simulink model "bdot_dynamic_test"  (R2016b)
settings: Solver=ode23tb  StartTime=0.0  StopTime=1000  RelTol=1e-3  EnableMultiTasking=on
libraries: dynamics_lib x1, environment_lib x1, bdot_controller_lib x1, command_processing x1, magnetometer_lib x1, magnetorquer_assembly_lib x1
settings Model: Creator=Taylor  LastModifiedBy=Taylor
settings OptimizationCC: DefaultParameterBehavior=Inlined  UseDivisionForNetSlopeComputation=on  UseFloatMulNetSlope=on  InlineInvariantSignals=on  PassReuseOutputArgsAs=Individual arguments  ZeroExternalMemoryAtStartup=off  ZeroInternalMemoryAtStartup=off  NoFixptDivByZeroProtection=on  EfficientFloat2IntCast=on  LifeSpan=1
settings DebuggingCC: ParameterTunabilityLossMsg=error  SFUnexpectedBacktrackingDiag=warning  SFNoUnconditionalDefaultTransitionDiag=warning  SFExecutionAtInitializationDiag=none
settings HardwareCC: ProdBitPerInt=16  ProdBitPerPointer=16  ProdBitPerSizeT=16  ProdBitPerPtrDiffT=16  ProdLargestAtomicFloat=None  ProdWordSize=16  ProdHWDeviceType=Texas Instruments->MSP430
settings RTWCC: SystemTargetFile=ert.tlc  TemplateMakefile=ert_default_tmf  Description=Embedded Coder  GenerateReport=on  IncludeHyperlinkInReport=on  LaunchReport=on  GenerateTraceInfo=on  GenerateTraceReport=on  GenerateTraceReportSl=on  GenerateTraceReportSf=on  GenerateTraceReportEml=on  GenerateCodeMetricsReport=on
settings CodeAppCC: ForceParamTrailComments=on  IgnoreCustomStorageClasses=off  OperatorAnnotations=on  SimulinkDataObjDesc=on  SFDataObjDesc=on  MATLABFcnDesc=on  CustomSymbolStrGlobalVar=rt$N$M  CustomSymbolStrType=$N$M  CustomSymbolStrFcn=$N$M$F  CustomSymbolStrMacro=$N$M  InsertBlockDesc=on  MATLABSourceComments=on
settings ERTTargetCC: GenerateSampleERTMain=on  CombineSignalStateStructs=on  SupportComplex=off  SupportContinuousTime=on  SupportNonInlinedSFcns=on  InlinedParameterPlacement=NonHierarchical  ERTCustomFileTemplate=example_file_process.tlc  ERTFilePackagingFormat=CompactWithDataFile
settings ConfigComp: CovMetricSettings=dw  CovHtmlReporting=on  CovSaveCumulativeToWorkspaceVar=on  CovSaveSingleToWorkspaceVar=on  CovExternalEMLEnable=off

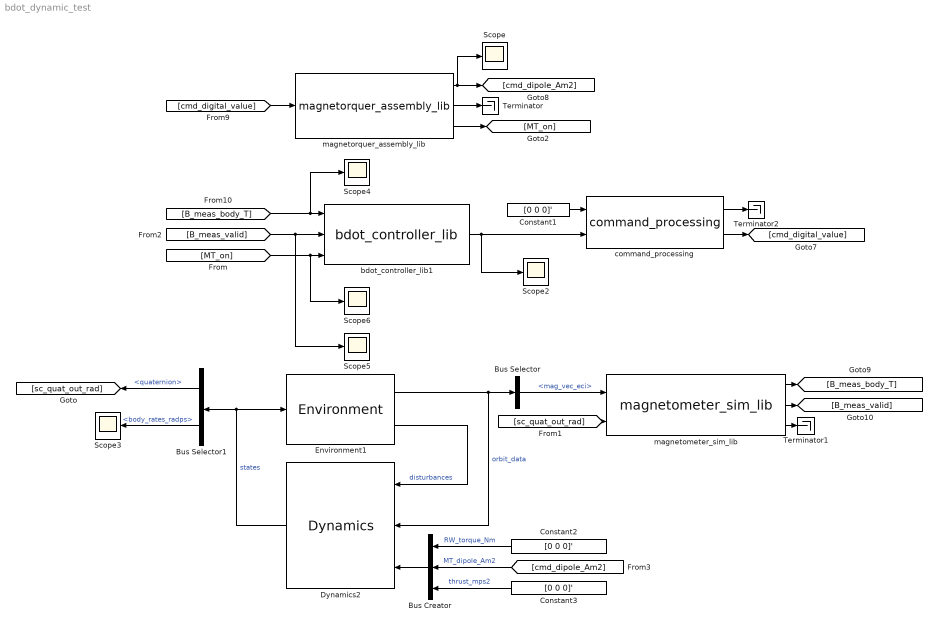
== system bdot_dynamic_test ==
  Bus Creator : BusCreator  Inputs=3
  Bus Selector : BusSelector  OutputSignals=mag_vec_eci
  Bus Selector1 : BusSelector  OutputSignals=quaternion,body_rates_radps
  Constant1 : Constant  Value=[0 0 0]'
  Constant2 : Constant  Value=[0 0 0]'
  Constant3 : Constant  Value=[0 0 0]'
  Dynamics2 : dynamics_lib/Dynamics
  Environment1 : environment_lib/Environment
  Scope{,2..6} (6 alike) : Scope
  Terminator : Terminator
  Terminator1 : Terminator
  Terminator2 : Terminator
  bdot_controller_lib1 : bdot_controller_lib/bdot_controller_lib
  command_processing : command_processing/command_processing
  magnetometer_sim_lib : magnetometer_lib/magnetometer_sim_lib
  magnetorquer_assembly_lib : magnetorquer_assembly_lib/magnetorquer_assembly_lib
  wires:
  bdot_controller_lib1/1 -> command_processing/2, Scope2/1
  [B_meas_body_T] -> Scope4/1, bdot_controller_lib1/1
  magnetometer_sim_lib/2 -> [B_meas_valid]
  magnetometer_sim_lib/1 -> [B_meas_body_T]
  magnetometer_sim_lib/3 -> Terminator1/1
  [sc_quat_out_rad] -> magnetometer_sim_lib/2
  [B_meas_valid] -> Scope5/1, bdot_controller_lib1/2
  [cmd_digital_value] -> magnetorquer_assembly_lib/1
  magnetorquer_assembly_lib/1 -> Scope/1, [cmd_dipole_Am2]
  magnetorquer_assembly_lib/2 -> Terminator/1
  magnetorquer_assembly_lib/3 -> [MT_on]
  [MT_on] -> Scope6/1, bdot_controller_lib1/3
  Environment1/1 -> Dynamics2/2, Bus Selector/1  "orbit_data"
  Environment1/2 -> Dynamics2/1  "disturbances"
  Bus Creator/1 -> Dynamics2/3
  Dynamics2/1 -> Bus Selector1/1, Environment1/1  "states"
  Constant2/1 -> Bus Creator/1  "RW_torque_Nm"
  [cmd_dipole_Am2] -> Bus Creator/2  "MT_dipole_Am2"
  Bus Selector/1 -> magnetometer_sim_lib/1  "<mag_vec_eci>"
  Bus Selector1/1 -> [sc_quat_out_rad]  "<quaternion>"
  Bus Selector1/2 -> Scope3/1  "<body_rates_radps>"
  Constant1/1 -> command_processing/1
  command_processing/2 -> [cmd_digital_value]
  command_processing/1 -> Terminator2/1
  Constant3/1 -> Bus Creator/3  "thrust_mps2"
